simulink model "smo"  (R2019b)
settings: Solver=ode4  StartTime=0.0  StopTime=inf  FixedStep=0.004  MaxStep=0.01  RelTol=1e-3
InitFcn:
  | [lowpass_B, lowpass_A] = butter(4,1,'s');
  | manipulator_tree = importrobot('description.urdf');
  | manipulator_tree.Gravity = [9.81 0 0];
model workspace (MAT data in the model file):
  SL_ROS_VariableLengthArrays_MaxSizes.CommonInfo.ArrayTruncateAction = 'EmitWarning'
  SL_ROS_VariableLengthArrays_MaxSizes.MsgTypeMap = containers.Map
  SL_ROS_VariableLengthArrays_MaxSizes.MsgTypeMap.serialization.keys = {'sensor_msgs/JointState', 'std_msgs/Float32MultiArray', 'std_msgs/Float64MultiArray', 'std_msgs/String'}
  SL_ROS_VariableLengthArrays_MaxSizes.MsgTypeMap.serialization.values{1}(1).PropertyName = 'Effort'
  SL_ROS_VariableLengthArrays_MaxSizes.MsgTypeMap.serialization.values{1}(1).DataType = 'double'
  SL_ROS_VariableLengthArrays_MaxSizes.MsgTypeMap.serialization.values{1}(1).MaxLength = 7
  SL_ROS_VariableLengthArrays_MaxSizes.MsgTypeMap.serialization.values{1}(2).PropertyName = 'Name'
  SL_ROS_VariableLengthArrays_MaxSizes.MsgTypeMap.serialization.values{1}(2).DataType = 'std_msgs/String'
  SL_ROS_VariableLengthArrays_MaxSizes.MsgTypeMap.serialization.values{1}(2).MaxLength = 7
  SL_ROS_VariableLengthArrays_MaxSizes.MsgTypeMap.serialization.values{1}(3).PropertyName = 'Position'
  SL_ROS_VariableLengthArrays_MaxSizes.MsgTypeMap.serialization.values{1}(3).DataType = 'double'
  SL_ROS_VariableLengthArrays_MaxSizes.MsgTypeMap.serialization.values{1}(3).MaxLength = 7
  SL_ROS_VariableLengthArrays_MaxSizes.MsgTypeMap.serialization.values{1}(4).PropertyName = 'Velocity'
  SL_ROS_VariableLengthArrays_MaxSizes.MsgTypeMap.serialization.values{1}(4).DataType = 'double'
  SL_ROS_VariableLengthArrays_MaxSizes.MsgTypeMap.serialization.values{1}(4).MaxLength = 7
  SL_ROS_VariableLengthArrays_MaxSizes.MsgTypeMap.serialization.values{2}.PropertyName = 'Data'
  SL_ROS_VariableLengthArrays_MaxSizes.MsgTypeMap.serialization.values{2}.DataType = 'single'
  SL_ROS_VariableLengthArrays_MaxSizes.MsgTypeMap.serialization.values{2}.MaxLength = 14
  SL_ROS_VariableLengthArrays_MaxSizes.MsgTypeMap.serialization.values{3}.PropertyName = 'Data'
  SL_ROS_VariableLengthArrays_MaxSizes.MsgTypeMap.serialization.values{3}.DataType = 'double'
  SL_ROS_VariableLengthArrays_MaxSizes.MsgTypeMap.serialization.values{3}.MaxLength = 7
  SL_ROS_VariableLengthArrays_MaxSizes.MsgTypeMap.serialization.values{4}.PropertyName = 'Data'
  SL_ROS_VariableLengthArrays_MaxSizes.MsgTypeMap.serialization.values{4}.DataType = 'uint8'
  SL_ROS_VariableLengthArrays_MaxSizes.MsgTypeMap.serialization.values{4}.MaxLength = 10
  SL_ROS_VariableLengthArrays_MaxSizes.MsgTypeMap.serialization.uniformity = 0
  SL_ROS_VariableLengthArrays_MaxSizes.MsgTypeMap.serialization.keyType = 'char'
  SL_ROS_VariableLengthArrays_MaxSizes.MsgTypeMap.serialization.valueType = 'any'
undefined symbols (not defined in the file or in its folder): Data, Data_SL_Info, lowpass_A, lowpass_B
libraries: robotlib x9, robotmaniplib x3, robotcorelib x1
settings Model: EnablePacing=on  Creator=marco  LastModifiedBy=marco
settings OptimizationCC: EnhancedBackFolding=on  PassReuseOutputArgsAs=Individual arguments  ZeroExternalMemoryAtStartup=off  ZeroInternalMemoryAtStartup=off  MaxStackSize=64  OptimizeBlockOrder=speed  DifferentSizesBufferReuse=on  OptimizationCustomize=off  EfficientTunableParamExpr=on
settings DebuggingCC: ParameterTunabilityLossMsg=error
settings HardwareCC: ProdBitPerLong=64  ProdHWDeviceType=Intel->x86-64 (Linux 64)
settings SFSimCC: CustomCodeUndefinedFunction=ThrowError
settings RTWCC: SystemTargetFile=ert.tlc  HardwareBoard=Robot Operating System (ROS)  TLCOptions="-aInlineSetEventsForThisBaseRateFcn=TLC_FALSE -aSuppressMultiTaskScheduler=TLC_FALSE  -aRateBasedStepFcn=0"  TemplateMakefile=ert_default_tmf  GenerateReport=on  Toolchain=Catkin  IncludeHyperlinkInReport=on  LaunchReport=on  TargetLang=C++  GenerateTraceInfo=on  GenerateTraceReport=on  GenerateTraceReportSl=on  GenerateTraceReportSf=on  GenerateTraceReportEml=on
settings CodeAppCC: ForceParamTrailComments=on  IgnoreCustomStorageClasses=off  OperatorAnnotations=on  SimulinkDataObjDesc=on  SFDataObjDesc=on  InsertBlockDesc=on
settings ERTTargetCC: SupportContinuousTime=on  SupportVariableSizeSignals=on
settings ExplorerConfigSet: InternalSimMechanicsExplorerSettings="<ExplorerConfiguration><canonicalview>aerospace</canonicalview><AnimationSetting><BasePlaybackSpeed>1.0</BasePlaybackSpeed><PlaybackSpeedFactor>1.0</PlaybackSpeedFactor></AnimationSetting><TilePanel><TileInfo><Tiles Columns=\"1\" Count=\"1\" Rows=\"1\"><Column Weight=\"1\"/><Row Weight=\"1\"/><Tile Height=\"1\" Width=\"1\" X=\"0\" Y=\"0\"/></Tiles></TileInfo><SceneInfo><SceneViewer><BGColor><R>0.60000002384185791</R><G>0.60000002384185791</G><B>0.60000002384185791</B></BGColor><Camera><DoPerspective>off</DoPerspective><Position><X>0.470747241724220999</X><Y>0.672742710715300452</Y><Z>0.803552756362765797</Z></Position><Center><X>0.426167977285198674</X><Y>0.0857009724355916047</Y><Z>-0.00477557216445684274</Z></Center><Up><X>-0.998971998504803671</X><Y>0.0328560329609175472</Y><Z>0.0312318315407420499</Z></Up><ViewLimDist>1</ViewLimDist><YLim>0.446111832261085528</YLim><XLim>0.664557689711664734</XLim></Camera></SceneViewer></SceneInfo></TilePanel><MechEditorPanel><Cameras/><GfxPanelCameraMap/><VideoCreator><PlaybackSpeedRatio>1.0</PlaybackSpeedRatio><FrameRate>30</FrameRate><VideoFormat>Motion JPEG AVI</VideoFormat><FrameSize>auto</FrameSize></VideoCreator></MechEditorPanel></ExplorerConfiguration>"

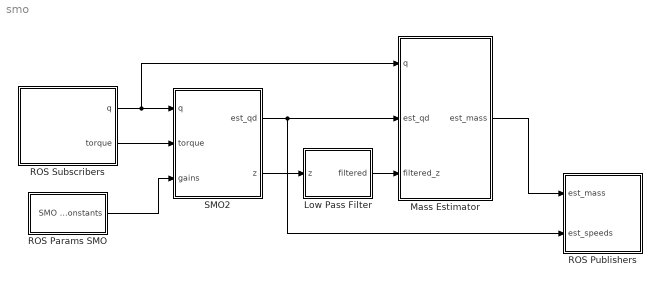
== system smo ==
  Low Pass Filter : Subsystem
  Mass Estimator : Subsystem
  ROS Params SMO : Subsystem
  ROS Publishers : Subsystem
  ROS Subscribers : Subsystem
  SMO2 : Subsystem
  wires:
  ROS Subscribers/1(q) -> Mass Estimator/1(q), SMO2/1(q)
  SMO2/1(est_qd) -> ROS Publishers/2("est_speeds "), Mass Estimator/2(est_qd)
  SMO2/2(z) -> Low Pass Filter/1(z)
  Low Pass Filter/1(filtered) -> Mass Estimator/3(filtered_z)
  Mass Estimator/1(est_mass) -> ROS Publishers/1(est_mass)
  ROS Params SMO/1(SMO Constants) -> SMO2/3(gains)
  ROS Subscribers/2(torque) -> SMO2/2(torque)

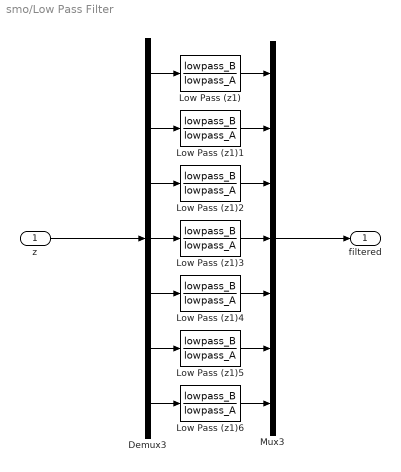
== system smo/Low Pass Filter ==
  z : Inport
  Demux3 : Demux  Outputs=7
  Low Pass (z1){,1..6} (7 alike) : TransferFcn  Numerator=lowpass_B  Denominator=lowpass_A
  Mux3 : Mux  Inputs=7
  filtered : Outport
  wires:
  Demux3/1 -> Low Pass (z1)/1
  Low Pass (z1)5/1 -> Mux3/6
  Low Pass (z1)2/1 -> Mux3/3
  Demux3/6 -> Low Pass (z1)5/1
  Low Pass (z1)4/1 -> Mux3/5
  z/1 -> Demux3/1
  Demux3/7 -> Low Pass (z1)6/1
  Demux3/5 -> Low Pass (z1)4/1
  Low Pass (z1)/1 -> Mux3/1
  Demux3/2 -> Low Pass (z1)1/1
  Mux3/1 -> filtered/1
  Low Pass (z1)6/1 -> Mux3/7
  Low Pass (z1)1/1 -> Mux3/2
  Demux3/4 -> Low Pass (z1)3/1
  Low Pass (z1)3/1 -> Mux3/4
  Demux3/3 -> Low Pass (z1)2/1

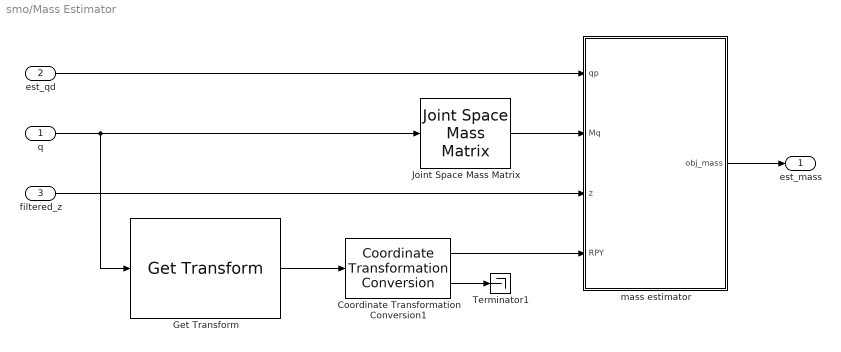
== system smo/Mass Estimator ==
  q : Inport
  est_qd : Inport  Port=2
  filtered_z : Inport  Port=3
  Coordinate Transformation Conversion1 : robotcorelib/Coordinate Transformation Conversion  InputRepresentation=Homogeneous Transformation  InputEulerSequence=ZYX  ShowTrVecInputPort=on  OutputRepresentation=Euler Angles  OutputEulerSequence=ZYX  ShowTrVecOutputPort=on  SimulateUsing=Code generation
      settings: SourceProductBaseCode=RO
  Get Transform : robotmaniplib/Get Transform  RigidBodyTree=manipulator_tree  SourceBody=shoulders_left_link  TargetBody=left_arm_link6  SimulateUsing=Code generation
      settings: SourceProductName=Robotics System Toolbox
  Joint Space Mass Matrix : robotmaniplib/Joint Space Mass Matrix  RigidBodyTree=manipulator_tree  SimulateUsing=Code generation
      settings: SourceProductName=Robotics System Toolbox
  Terminator1 : Terminator
  mass estimator : MATLAB Function  TreatAsAtomicUnit=on
  est_mass : Outport
  wires:
  Get Transform/1 -> Coordinate Transformation Conversion1/1
  Joint Space Mass Matrix/1 -> mass estimator/2(Mq)
  q/1 -> Get Transform/1, Joint Space Mass Matrix/1
  mass estimator/1(obj_mass) -> est_mass/1
  est_qd/1 -> mass estimator/1(qp)
  filtered_z/1 -> mass estimator/3(z)
  Coordinate Transformation Conversion1/2 -> Terminator1/1
  Coordinate Transformation Conversion1/1 -> mass estimator/4(RPY)

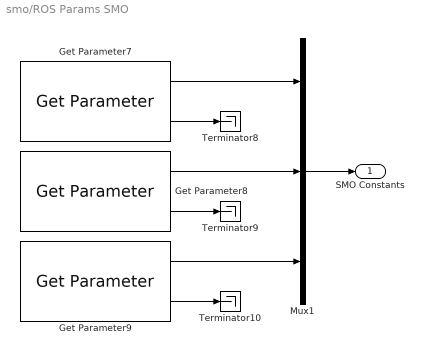
== system smo/ROS Params SMO ==
  Get Parameter7 : robotlib/Get Parameter  ParameterSource=Specify your own  ParameterName=/smo/lambda  ParameterType=double  ParameterMaxArrayLength=16  ParameterInitialValue=0.0  SampleTime=1  ShowErrorCodeOutput=on  ModelName=smo  BlockId=ParamGet_smo_383
      settings: SourceProductName=ROS Toolbox  SourceProductBaseCode=RR
  Get Parameter8 : robotlib/Get Parameter  ParameterSource=Specify your own  ParameterName=/smo/alpha  ParameterType=double  ParameterMaxArrayLength=16  ParameterInitialValue=0.0  SampleTime=1  ShowErrorCodeOutput=on  ModelName=smo  BlockId=ParamGet_smo_384
      settings: SourceProductName=ROS Toolbox  SourceProductBaseCode=RR
  Get Parameter9 : robotlib/Get Parameter  ParameterSource=Specify your own  ParameterName=/smo/gamma  ParameterType=double  ParameterMaxArrayLength=16  ParameterInitialValue=0.0  SampleTime=1  ShowErrorCodeOutput=on  ModelName=smo  BlockId=ParamGet_smo_385
      settings: SourceProductName=ROS Toolbox  SourceProductBaseCode=RR
  Mux1 : Mux  Inputs=3
  Terminator10 : Terminator
  Terminator8 : Terminator
  Terminator9 : Terminator
  SMO Constants : Outport
  wires:
  Get Parameter9/1 -> Mux1/3
  Get Parameter7/1 -> Mux1/1
  Get Parameter7/2 -> Terminator8/1
  Mux1/1 -> SMO Constants/1
  Get Parameter8/2 -> Terminator9/1
  Get Parameter9/2 -> Terminator10/1
  Get Parameter8/1 -> Mux1/2

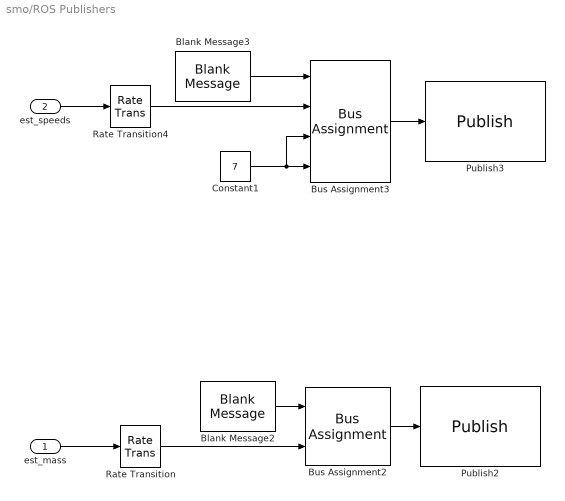
== system smo/ROS Publishers ==
  est_mass : Inport
  "est_speeds " : Inport  Port=2
  Blank Message2 : robotlib/Blank Message  messageClass=Message  entityType=std_msgs/Float64  messageType=std_msgs/Float64  SampleTime=0.04
      settings: SourceProductName=ROS Toolbox
  Blank Message3 : robotlib/Blank Message  messageClass=Message  entityType=std_msgs/Float64MultiArray  messageType=std_msgs/Float64MultiArray  SampleTime=0.004
      settings: SourceProductName=ROS Toolbox
  Bus Assignment2 : BusAssignment  AssignedSignals=Data
  Bus Assignment3 : BusAssignment  AssignedSignals=Data,Data_SL_Info.CurrentLength,Data_SL_Info.ReceivedLength
  Constant1 : Constant  Value=7  OutDataTypeStr=uint32  SampleTime=0.004
  Publish2 : robotlib/Publish  topicSource=Specify your own  topic=/estimated_mass  messageType=std_msgs/Float64  messageQueueLength=1
      settings: SourceProductName=ROS Toolbox
  Publish3 : robotlib/Publish  topicSource=Specify your own  topic=/smo/estimated_speeds  messageType=std_msgs/Float64MultiArray  messageQueueLength=1
      settings: SourceProductName=ROS Toolbox
  Rate Transition : RateTransition
  Rate Transition4 : RateTransition
  wires:
  Blank Message2/1 -> Bus Assignment2/1
  Rate Transition/1 -> Bus Assignment2/2
  Bus Assignment2/1 -> Publish2/1
  Rate Transition4/1 -> Bus Assignment3/2
  Bus Assignment3/1 -> Publish3/1
  Constant1/1 -> Bus Assignment3/4, Bus Assignment3/3
  Blank Message3/1 -> Bus Assignment3/1
  est_mass/1 -> Rate Transition/1
  "est_speeds "/1 -> Rate Transition4/1

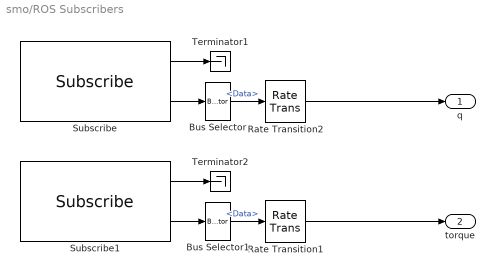
== system smo/ROS Subscribers ==
  Bus Selector : BusSelector  OutputSignals=Data
  Bus Selector1 : BusSelector  OutputSignals=Data
  Rate Transition1 : RateTransition
  Rate Transition2 : RateTransition
  Subscribe : robotlib/Subscribe  topicSource=Specify your own  topic=/joint_positions  messageType=std_msgs/Float64MultiArray  sampleTime=0.004  messageQueueLength=1
      settings: SourceProductName=ROS Toolbox
  Subscribe1 : robotlib/Subscribe  topicSource=Specify your own  topic=/joint_torques  messageType=std_msgs/Float64MultiArray  sampleTime=0.004  messageQueueLength=1
      settings: SourceProductName=ROS Toolbox
  Terminator1 : Terminator
  Terminator2 : Terminator
  q : Outport
  torque : Outport  Port=2
  wires:
  Bus Selector/1 -> Rate Transition2/1  "<Data>"
  Rate Transition2/1 -> q/1
  Subscribe/2 -> Bus Selector/1
  Subscribe/1 -> Terminator1/1
  Subscribe1/1 -> Terminator2/1
  Subscribe1/2 -> Bus Selector1/1
  Bus Selector1/1 -> Rate Transition1/1  "<Data>"
  Rate Transition1/1 -> torque/1

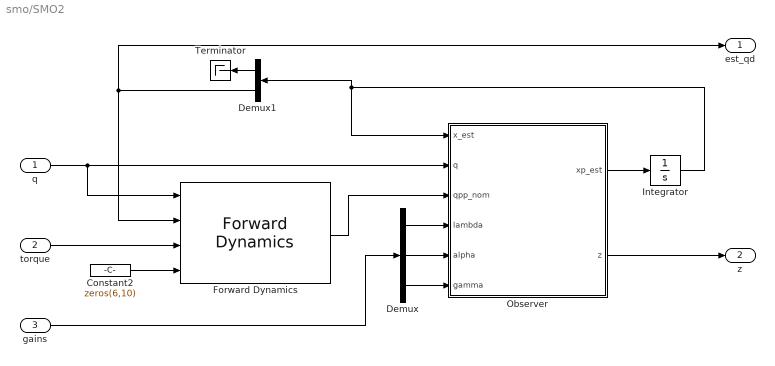
== system smo/SMO2 ==
  q : Inport
  torque : Inport  Port=2
  gains : Inport  Port=3
  Constant2 : Constant  Value=zeros(6,10)  SampleTime=-1
  Demux : Demux  Outputs=3
  Demux1 : Demux  Outputs=[7,7]
  Forward Dynamics : robotmaniplib/Forward Dynamics  RigidBodyTree=manipulator_tree  SimulateUsing=Code generation
      settings: SourceProductName=Robotics System Toolbox
  Integrator : Integrator  InitialCondition=[0 0 0 0 0 0 0 0 0 0 0 0 0 0]
  Observer : MATLAB Function  TreatAsAtomicUnit=on
  Terminator : Terminator
  est_qd : Outport
  z : Outport  Port=2
  wires:
  gains/1 -> Demux/1
  Demux/1 -> Observer/4(lambda)
  Demux/2 -> Observer/5(alpha)
  Demux/3 -> Observer/6(gamma)
  Demux1/2 -> Forward Dynamics/2, est_qd/1
  q/1 -> Observer/2(q), Forward Dynamics/1
  Observer/2(z) -> z/1
  torque/1 -> Forward Dynamics/3
  Integrator/1 -> Observer/1(x_est), Demux1/1
  Forward Dynamics/1 -> Observer/3(qpp_nom)
  Observer/1(xp_est) -> Integrator/1
  Demux1/1 -> Terminator/1
  Constant2/1 -> Forward Dynamics/4

== matlab function smo/Mass Estimator/mass estimator ==
  data: qp input; Mq input; z input; RPY input; obj_mass output
function obj_mass = mass_est(qp, Mq, z, RPY)
phi = Mq*z;
g = 9.81;
l = 0.21;
vel = norm(qp);
pitch = RPY(2);

%obj_mass = phi(6)/l/g;
if abs(sin(pitch)) > 0.2 && vel < 0.15
    obj_mass = -phi(6)/(l*g*sin(pitch));
else
    obj_mass = 0;
end

% function obj_mass = mass_est(q, qp, z, Mq)
% phi = Mq*z;
% g = 9.81;
% l = 0.195;
% vel = norm(qp);
% %obj_mass = zeros(1,2);
% if abs(sin(q(1) + q(4) + q(6))) > 0.1 && vel < 0.1
%     obj_mass = -phi(6)/(l*g*sin(q(1) + q(4) + q(6)));
%     %obj_mass(2) = -phi(4)/(0.33*9.81*sin(q(1) + q(4)));
% else
%     obj_mass = 0;
% end

== matlab function smo/SMO2/Observer ==
  data: x_est input; q input; qpp_nom input; xp_est output; z output; lambda input; alpha input; gamma input
function [xp_est, z] = observer(x_est, q, qpp_nom, lambda, alpha, gamma)
xp_est = zeros(1,14);
q_est  = x_est(1:7);
qp_est = x_est(8:14);
z1 = zeros(1,7);
z2 = zeros(1,7);

%lambda = 10;
%alpha  = 10;
%lambda = 6;
%alpha  = 4.2;
%gamma = 0.001;

for i=1:7
    %z1(i) = lambda*sqrt(abs(q(i) - q_est(i)))*sign(q(i) - q_est(i));
    %z2(i) = alpha*sign(q(i) - q_est(i));
    z1(i) = lambda*sqrt(abs(q(i) - q_est(i)))*(2/(1 + exp((q_est(i) - q(i))/gamma)) - 1);
    z2(i) = alpha*(2/(1 + exp((q_est(i) - q(i))/gamma)) - 1);
end

for i=1:7
    xp_est(i)   = qp_est(i) + z1(i);
    xp_est(i+7) = qpp_nom(i) + z2(i);
end

z = z2;
